simulink model "vpc_new_ut"  (Simulink 8.1)
settings: Solver=FixedStepDiscrete  StartTime=0.0  StopTime=10.0  FixedStep=5E-3  RelTol=1e-3
libraries: siltestlib x10, idiada_lib x9, vpc_new x1
settings Model: Creator=xsellart  LastModifiedBy=AT015555
settings DataIOCC: SignalLoggingSaveFormat=Dataset
settings OptimizationCC: ExpressionDepthLimit=128
settings DebuggingCC: FcnCallInpInsideContextMsg=EnableAllAsError
settings GRTTargetCC: CombineOutputUpdateFcns=on  GRTInterface=off

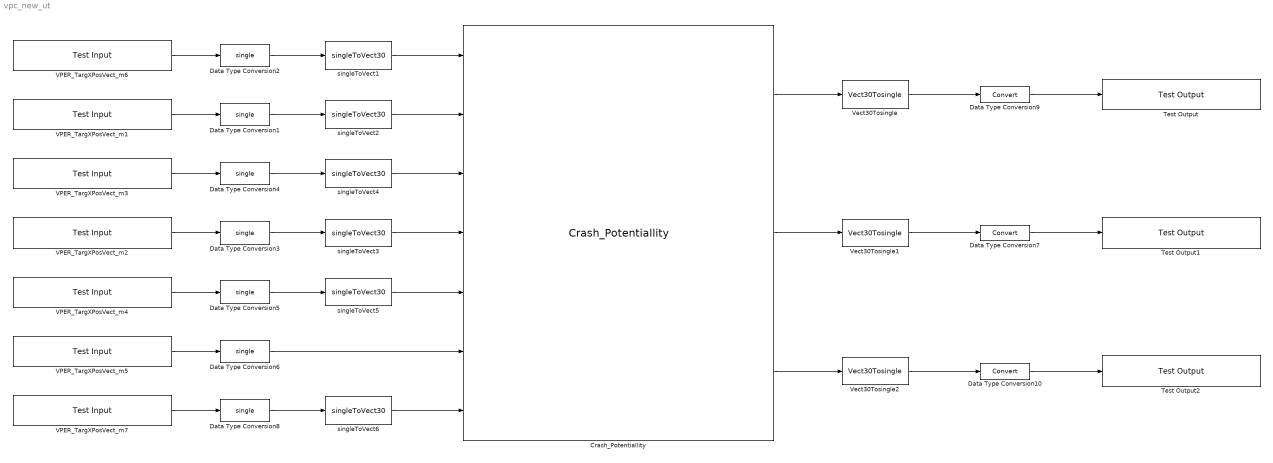
== system vpc_new_ut ==
  Crash_Potentiallity : vpc_new/Crash_Potentiallity
  Data Type Conversion{1..6,8} (7 alike) : DataTypeConversion  OutDataTypeStr=single
  Data Type Conversion10 : DataTypeConversion
  Data Type Conversion7 : DataTypeConversion
  Data Type Conversion9 : DataTypeConversion
  Test Output : siltestlib/Test Output  varname=VIFO_VRUIsPotentialVect30_flg  sampletime=-1
  Test Output1 : siltestlib/Test Output  varname=VIFO_SimpleTTCxVect30_s  sampletime=-1
  Test Output2 : siltestlib/Test Output  varname=VIFO_PotentiallityVect30_perc  sampletime=-1
  VPER_TargXPosVect_m1 : siltestlib/Test Input  varname=VIFO_TargAbsSpeedYVect30_mps  sampletime=0.005
  VPER_TargXPosVect_m2 : siltestlib/Test Input  varname=VIFO_TargVehRelSpeedXVect30_mps  sampletime=0.005
  VPER_TargXPosVect_m3 : siltestlib/Test Input  varname=VPER_TargXPosVect30_m  sampletime=0.005
  VPER_TargXPosVect_m4 : siltestlib/Test Input  varname=VPER_TargIdVect30_num  sampletime=0.005
  VPER_TargXPosVect_m5 : siltestlib/Test Input  varname=VPER_NumberOfTargets_enum  sampletime=0.005
  VPER_TargXPosVect_m6 : siltestlib/Test Input  varname=VPER_TargYPosVect30_m  sampletime=0.005
  VPER_TargXPosVect_m7 : siltestlib/Test Input  varname=VIFO_AEBVehInPathVect30_flg  sampletime=0.005
  Vect30Tosingle : idiada_lib/Vect30Tosingle
  Vect30Tosingle1 : idiada_lib/Vect30Tosingle
  Vect30Tosingle2 : idiada_lib/Vect30Tosingle
  singleToVect{1..6} (6 alike) : idiada_lib/singleToVect30
  wires:
  VPER_TargXPosVect_m6/1 -> Data Type Conversion2/1
  Data Type Conversion2/1 -> singleToVect1/1
  VPER_TargXPosVect_m1/1 -> Data Type Conversion1/1
  Data Type Conversion1/1 -> singleToVect2/1
  VPER_TargXPosVect_m2/1 -> Data Type Conversion3/1
  Data Type Conversion3/1 -> singleToVect3/1
  VPER_TargXPosVect_m3/1 -> Data Type Conversion4/1
  Data Type Conversion4/1 -> singleToVect4/1
  VPER_TargXPosVect_m4/1 -> Data Type Conversion5/1
  Data Type Conversion5/1 -> singleToVect5/1
  VPER_TargXPosVect_m5/1 -> Data Type Conversion6/1
  VPER_TargXPosVect_m7/1 -> Data Type Conversion8/1
  Data Type Conversion8/1 -> singleToVect6/1
  Data Type Conversion6/1 -> Crash_Potentiallity/6
  singleToVect6/1 -> Crash_Potentiallity/7
  singleToVect4/1 -> Crash_Potentiallity/3
  singleToVect2/1 -> Crash_Potentiallity/2
  singleToVect5/1 -> Crash_Potentiallity/5
  singleToVect3/1 -> Crash_Potentiallity/4
  singleToVect1/1 -> Crash_Potentiallity/1
  Crash_Potentiallity/1 -> Vect30Tosingle/1
  Data Type Conversion9/1 -> Test Output/1
  Vect30Tosingle/1 -> Data Type Conversion9/1
  Data Type Conversion7/1 -> Test Output1/1
  Vect30Tosingle1/1 -> Data Type Conversion7/1
  Data Type Conversion10/1 -> Test Output2/1
  Vect30Tosingle2/1 -> Data Type Conversion10/1
  Crash_Potentiallity/2 -> Vect30Tosingle1/1
  Crash_Potentiallity/3 -> Vect30Tosingle2/1
